simulink model "aeroblk_wf_3dof_noVR"  (Simulink 6.0)
settings: Solver=ode45  StartTime=0.0  StopTime=10  FixedStep=0.01  MaxStep=0.02  RelTol=1e-3
PreLoadFcn:
  | aeroblk_wf_3dof_data;
libraries: aeroblk_lib_wf_3dof x3, simulink x1
CloseFcn:
  | clear wf_B3 wf_H wf_Q2 wf_Q4 wf_alpha wf_alpha2 wf_alphaa wf_c wf_cd wf_cg wf_cl wf_cls wf_cm wf_cp_e wf_gravity wf_incidence wf_weight wf_z1 wf_z2 wf_z3 wf_inertia wf_sref wf_w2e wf_q;
  | 
  | clear ports tempFixPtSimRanges
settings Model: Creator=The MathWorks Inc.  LastModifiedBy=batserve  ExtModeAutoUpdateStatusClock=off
settings DataIOCC: SaveOutput=off  SaveTime=off  SignalLoggingName=sigsOut
settings OptimizationCC: InlineInvariantSignals=off
settings DebuggingCC: CheckExecutionContextPreStartOutputMsg=on  CheckExecutionContextRuntimeOutputMsg=on  SolverPrmCheckMsg=none
settings HardwareCC: TargetUnknown=on

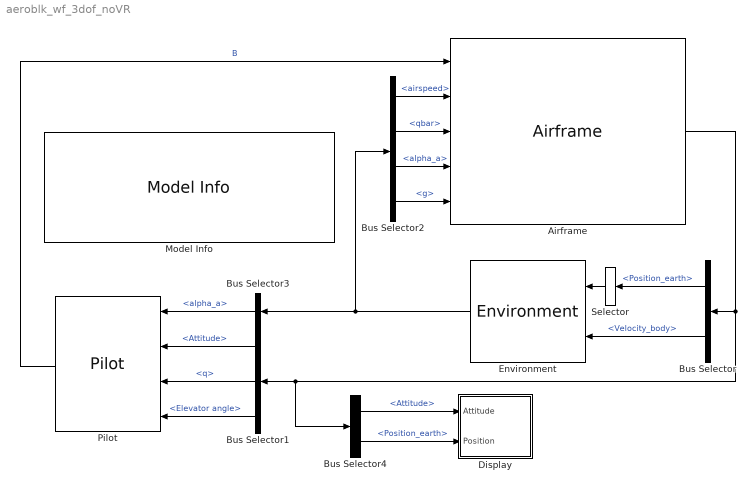
== system aeroblk_wf_3dof_noVR ==
  Airframe : aeroblk_lib_wf_3dof/Airframe
  Bus Selector : BusSelector  Orientation=left  DialogController=Simulink.DDGSource_Bus  OutputSignals=Position_earth,Velocity_body
  Bus Selector1 : BusSelector  Orientation=left  DialogController=Simulink.DDGSource_Bus  OutputSignals=Attitude,q,Elevator angle
  Bus Selector2 : BusSelector  DialogController=Simulink.DDGSource_Bus  OutputSignals=airspeed,qbar,alpha_a,g
  Bus Selector3 : BusSelector  Orientation=left  DialogController=Simulink.DDGSource_Bus  OutputSignals=alpha_a
  Bus Selector4 : BusSelector  DialogController=Simulink.DDGSource_Bus  OutputSignals=Attitude,Position_earth
  Display : Subsystem  PropExecContextAcrossSSBoundary=on
      mask Display:
      | port_label('input',1,'Altitude')
      | port_label('input',2,'Position')
  Environment : aeroblk_lib_wf_3dof/Environment  Orientation=left
  Model Info : simulink/Model-Wide Utilities/Model Info  InitialBlockCM=None  BlockCM=None  Frame=on  DisplayStringWithTags=|  HorizontalTextAlignment=Center  LeftAlignmentValue=0.5  SourceBlockDiagram=aeroblk_wf_3dof_noVR  TagMaxNumber=20
      | 1903 Wright Flyer
      | based on 
      | Hooven, Frederick J., "Longitudinal 
      | Dynamics of the Wright Brothers' Early Flyers 
      | 'A Study in Computer Simulation of Flight'", 
      | from The Wright Flyer An Engineering Perspective 
      | edited by Howard S. Wolko, 1987.%<Description>
  Pilot : aeroblk_lib_wf_3dof/Pilot  Orientation=left
  Selector : Selector  Orientation=left  Elements=2  InputPortWidth=2
  wires:
  Environment/1 -> Bus Selector2/1, Bus Selector3/1
  Pilot/1 -> Airframe/1  "B"
  Airframe/1 -> Bus Selector/1, Bus Selector1/1, Bus Selector4/1
  Bus Selector/1 -> Selector/1  "<Position_earth>"
  Bus Selector/2 -> Environment/2  "<Velocity_body>"
  Selector/1 -> Environment/1
  Bus Selector1/1 -> Pilot/2  "<Attitude>"
  Bus Selector1/2 -> Pilot/3  "<q>"
  Bus Selector1/3 -> Pilot/4  "<Elevator angle>"
  Bus Selector2/1 -> Airframe/2  "<airspeed>"
  Bus Selector2/2 -> Airframe/3  "<qbar>"
  Bus Selector2/3 -> Airframe/4  "<alpha_a>"
  Bus Selector2/4 -> Airframe/5  "<g>"
  Bus Selector3/1 -> Pilot/1  "<alpha_a>"
  Bus Selector4/2 -> Display/2(Position)  "<Position_earth>"
  Bus Selector4/1 -> Display/1(Attitude)  "<Attitude>"

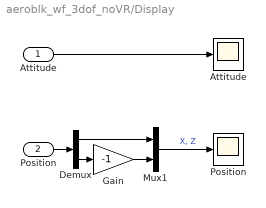
== system aeroblk_wf_3dof_noVR/Display ==
  Attitude : Inport  Port=1  LatchInput=off
  Position : Inport  Port=2  LatchInput=off
  "Attitude " : Scope
      settings: TimeRange=3  YMin=-0.16  YMax=-0.06
  Demux : Demux  Outputs=2
  Gain : Gain  Gain=-1  SaturateOnIntegerOverflow=on
  Mux1 : Mux  Inputs=2
  "Position " : Scope
      settings: TimeRange=3  YMin=-20  YMax=100
  wires:
  Attitude/1 -> "Attitude "/1
  Position/1 -> Demux/1
  Mux1/1 -> "Position "/1  "X, Z"
  Demux/2 -> Gain/1
  Gain/1 -> Mux1/2
  Demux/1 -> Mux1/1
